simulink model "project_model_UPDATE"  (R2020a)
settings: Solver=FixedStepAuto  StartTime=0.0  StopTime=10.0  FixedStep=1e-3  RelTol=1e-3  EnableMultiTasking=on
undefined symbols (not defined in the file): D0, D1, D10, D11, D12, D13, D2, D3, D4, D5, D6, D7, D8, D9, PTA0, PTA1, PTA2, PTB23, PTB9, PTC16, PTC17, PTC2, PTC3, PTC4, PTD0, PTD1, PTD2, PTD3
libraries: frdmk64flib x15
settings Model: ExtModeTrigDuration=5  Creator=harry  LastModifiedBy=harry
settings OptimizationCC: EnhancedBackFolding=on  PassReuseOutputArgsAs=Individual arguments  ZeroExternalMemoryAtStartup=off  ZeroInternalMemoryAtStartup=off  MaxStackSize=64  OptimizeBlockOrder=speed  DifferentSizesBufferReuse=on  OptimizationCustomize=off  EfficientTunableParamExpr=on
settings DebuggingCC: ParameterTunabilityLossMsg=error  UnconnectedInputMsg=none  UnconnectedOutputMsg=none  UnconnectedLineMsg=none  SFMachineParentedDataDiag=error
settings HardwareCC: ProdBitPerPointer=32  ProdBitPerSizeT=32  ProdBitPerPtrDiffT=32  ProdLargestAtomicInteger=Long  ProdLargestAtomicFloat=Double  ProdWordSize=32  ProdHWDeviceType=ARM Compatible->ARM Cortex
settings SFSimCC: MATLABDynamicMemAlloc=off
settings RTWCC: SystemTargetFile=ert.tlc  HardwareBoard=NXP FRDM-K64F  TemplateMakefile=ert_default_tmf  Toolchain=GNU Tools for ARM Embedded Processors
settings CodeAppCC: ForceParamTrailComments=on  IgnoreCustomStorageClasses=off  OperatorAnnotations=on  SimulinkDataObjDesc=on  SFDataObjDesc=on  InsertBlockDesc=on
settings ERTTargetCC: ExtModeTransport=4  ExtModeMexFile=sendToCommService

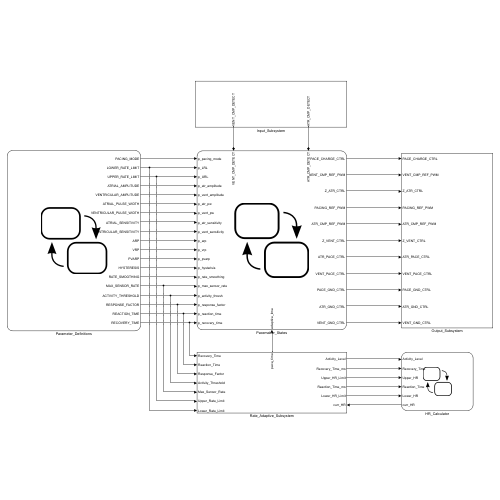
[thumbnail: Simulink's stored preview of the top-level diagram]
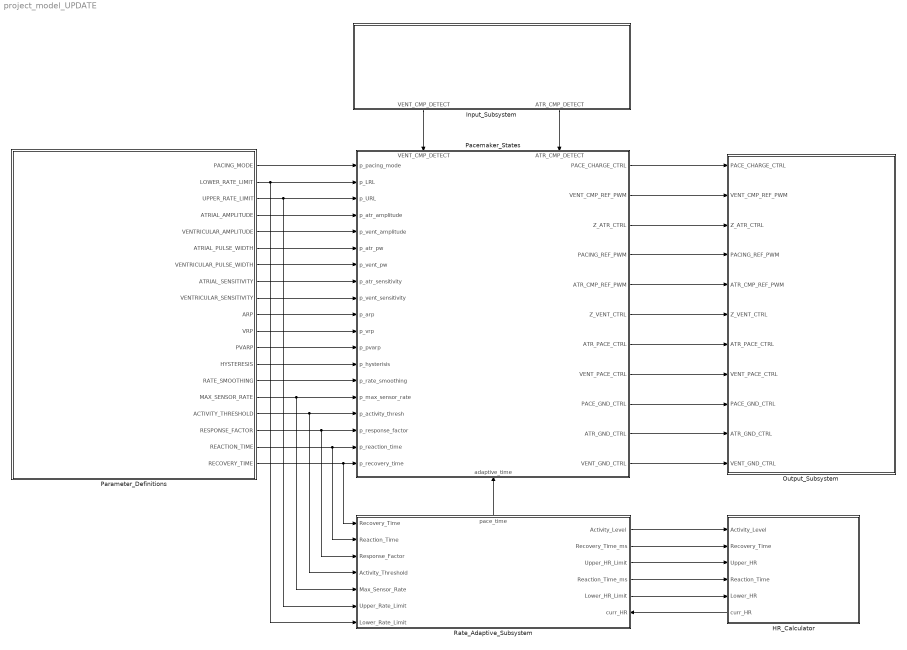
== system project_model_UPDATE ==
  HR_Calculator : Stateflow chart  TreatAsAtomicUnit=on
      settings: PortSchema="{\"entries\":[{\"content\":{\"sides\":[{\"content\":{\"connectorIds\":[\"In5\",\"In2\",\"In3\",\"In4\",\"In1\",\"Out1\"]},\"type\":\"ConnectorPlacement.EquallySpacedRectSide\",\"uuid\":\"4fd71a97-0d96-44cf-9a3b-b475d577ae04\"},{\"content\":{\"connectorIds\":[],\"side\":\"RIGHT\"},\"type\":\"ConnectorPlacement.EquallySpacedRectSide\",\"uuid\":\"faba256d-fac9-4ab5-bd75-12f2978d4ab7\"},{\"content\":{\"connectorIds\":[],\"side\":\"TOP\"},\"type\":\"ConnectorPlacement.EquallySpacedRectSide\",\"uuid\":\"a02d704a-be11-4cb0-b416-0f22440acd8a\"}]},\"type\":\"ConnectorPlacement.EquallySpacedConnector\",\"uuid\":\"fcc24184-24f4-4090-bbbe-791745e2298d\"}],\"packageUris\":[\"http://schema.mathworks.com/mf0/Connector/R2020b\"],\"version\":\"1.0\"}"
  Input_Subsystem : Subsystem
      settings: PortSchema="{\"entries\":[{\"content\":{\"sides\":[{\"content\":{\"connectorIds\":[]},\"type\":\"ConnectorPlacement.EquallySpacedRectSide\",\"uuid\":\"7aa35272-78af-4b86-b792-d4552822e5cd\"},{\"content\":{\"connectorIds\":[],\"side\":\"RIGHT\"},\"type\":\"ConnectorPlacement.EquallySpacedRectSide\",\"uuid\":\"1eeedbdd-e182-4d72-ab10-92c9b2e47973\"},{\"content\":{\"connectorIds\":[],\"side\":\"TOP\"},\"type\":\"ConnectorPlacement.EquallySpacedRectSide\",\"uuid\":\"983587ba-d25a-459a-9a3e-9f5267716506\"},{\"content\":{\"connectorIds\":[\"Out1\",\"Out2\"],\"side\":\"BOTTOM\"},\"type\":\"ConnectorPlacement.EquallySpacedRectSide\",\"uuid\":\"0cdd1530-a104-439a-8a9c-6ed3bc5e5b37\"}]},\"type\":\"ConnectorPlacement.EquallySpacedConnector\",\"uuid\":\"2c1020c0-9cac-4181-8f0f-8201f6fe3f1b\"}],\"packageUris\":[\"http://schema.mathworks.com/mf0/Connector/R2020b\"],\"version\":\"1.0\"}"
  Output_Subsystem : Subsystem
  Pacemaker_States : Stateflow chart  TreatAsAtomicUnit=on
      settings: PortSchema="{\"entries\":[{\"content\":{\"sides\":[{\"content\":{\"connectorIds\":[\"In9\",\"In5\",\"In15\",\"In7\",\"In4\",\"In8\",\"In6\",\"In13\",\"In14\",\"In11\",\"In12\",\"In17\",\"In10\",\"In16\",\"In18\",\"In19\",\"In20\",\"In22\",\"In21\"]},\"type\":\"ConnectorPlacement.EquallySpacedRectSide\",\"uuid\":\"f7c19d4e-8469-492c-a227-d3ddaf8b11c5\"},{\"content\":{\"connectorIds\":[\"Out8\",\"Out10\",\"Out1\",\"Out7\",\"Out11\",\"Out2\",\"Out3\",\"Out4\",\"Out9\",\"Out5\",\"Out6\"],\"side\":\"RIGHT\"},\"type\":\"ConnectorPlacement.EquallySpacedRectSide\",\"uuid\":\"dec5cef5-f41f-4673-aab9-f0ca8e60eeee\"},{\"content\":{\"connectorIds\":[\"In2\",\"In3\"],\"side\":\"TOP\"},\"type\":\"ConnectorPlacement.EquallySpacedRectSide\",\"uuid\":\"d69c500f-a27d-47d0-a981-29ab2c08cb35\"},{\"content\":{\"connectorIds\":[\"In1\"],\"side\":\"BOTTOM\"},\"type\":\"ConnectorPlacement.EquallySpacedRectSide\",\"uuid\":\"de5bd18b-94e5-479b-a57c-c3af68974efa\"}]},\"type\":\"ConnectorPlacement.EquallySpacedConnector\",\"uuid\":\"10b708de-b80e-4994-a949-6ddae67c2dfd\"}],\"packageUris\":[\"http://schema.mathworks.com/mf0/Connector/R2020b\"],\"version\":\"1.0\"}"
  Parameter_Definitions : Stateflow chart  TreatAsAtomicUnit=on
      settings: PortSchema="{\"entries\":[{\"content\":{\"sides\":[{\"content\":{\"connectorIds\":[]},\"type\":\"ConnectorPlacement.EquallySpacedRectSide\",\"uuid\":\"6604c324-2550-41c6-b2f2-71f3c706ced3\"},{\"content\":{\"connectorIds\":[\"Out1\",\"Out2\",\"Out3\",\"Out4\",\"Out7\",\"Out5\",\"Out9\",\"Out8\",\"Out6\",\"Out14\",\"Out13\",\"Out12\",\"Out11\",\"Out10\",\"Out16\",\"Out19\",\"Out15\",\"Out17\",\"Out18\"],\"side\":\"RIGHT\"},\"type\":\"ConnectorPlacement.EquallySpacedRectSide\",\"uuid\":\"7ef386a9-7013-4033-b302-df52cb7a11b5\"},{\"content\":{\"connectorIds\":[],\"side\":\"TOP\"},\"type\":\"ConnectorPlacement.EquallySpacedRectSide\",\"uuid\":\"6c75a8fc-d552-4f9b-9a9a-6aef7cb72f4d\"}]},\"type\":\"ConnectorPlacement.EquallySpacedConnector\",\"uuid\":\"c0dbf2bf-9097-47f1-93b4-de483c75bb4c\"}],\"packageUris\":[\"http://schema.mathworks.com/mf0/Connector/R2020b\"],\"version\":\"1.0\"}"
  Rate_Adaptive_Subsystem : Subsystem
      settings: PortSchema="{\"entries\":[{\"content\":{\"sides\":[{\"content\":{\"connectorIds\":[\"In1\",\"In2\",\"In3\",\"In4\",\"In5\",\"In6\",\"In7\"]},\"type\":\"ConnectorPlacement.EquallySpacedRectSide\",\"uuid\":\"0e73cd95-fd23-47fa-82ad-61e0ef758ad8\"},{\"content\":{\"connectorIds\":[\"Out1\",\"Out2\",\"Out3\",\"Out4\",\"Out5\",\"In8\"],\"side\":\"RIGHT\"},\"type\":\"ConnectorPlacement.EquallySpacedRectSide\",\"uuid\":\"257d0885-109f-47f8-9bd4-99d2095959ba\"},{\"content\":{\"connectorIds\":[\"Out6\"],\"side\":\"TOP\"},\"type\":\"ConnectorPlacement.EquallySpacedRectSide\",\"uuid\":\"5fbd8ae3-cd68-4bdc-a329-22cd7db730ea\"}]},\"type\":\"ConnectorPlacement.EquallySpacedConnector\",\"uuid\":\"229e8082-3f61-43cc-9449-39b4152275b7\"}],\"packageUris\":[\"http://schema.mathworks.com/mf0/Connector/R2020b\"],\"version\":\"1.0\"}"
  wires:
  Parameter_Definitions/10(RATE_SMOOTHING) -> Pacemaker_States/16(p_rate_smoothing)
  Parameter_Definitions/2(LOWER_RATE_LIMIT) -> Rate_Adaptive_Subsystem/7(Lower_Rate_Limit), Pacemaker_States/5(p_LRL)
  Rate_Adaptive_Subsystem/5(Lower_HR_Limit) -> HR_Calculator/1(Lower_HR)
  Parameter_Definitions/18(RECOVERY_TIME) -> Rate_Adaptive_Subsystem/1(Recovery_Time), Pacemaker_States/21(p_recovery_time)
  Pacemaker_States/9(PACE_GND_CTRL) -> Output_Subsystem/9(PACE_GND_CTRL)
  Parameter_Definitions/14(ARP) -> Pacemaker_States/11(p_arp)
  Pacemaker_States/5(ATR_GND_CTRL) -> Output_Subsystem/10(ATR_GND_CTRL)
  Pacemaker_States/10(VENT_CMP_REF_PWM) -> Output_Subsystem/2(VENT_CMP_REF_PWM)
  Pacemaker_States/6(VENT_GND_CTRL) -> Output_Subsystem/11(VENT_GND_CTRL)
  Parameter_Definitions/11(HYSTERESIS) -> Pacemaker_States/10(p_hysterisis)
  Rate_Adaptive_Subsystem/2(Recovery_Time_ms) -> HR_Calculator/2(Recovery_Time)
  Input_Subsystem/1(VENT_CMP_DETECT) -> Pacemaker_States/2(VENT_CMP_DETECT)
  Rate_Adaptive_Subsystem/6(pace_time) -> Pacemaker_States/1(adaptive_time)
  HR_Calculator/1(curr_HR) -> Rate_Adaptive_Subsystem/8(curr_HR)
  Input_Subsystem/2(ATR_CMP_DETECT) -> Pacemaker_States/3(ATR_CMP_DETECT)
  Pacemaker_States/8(PACE_CHARGE_CTRL) -> Output_Subsystem/1(PACE_CHARGE_CTRL)
  Rate_Adaptive_Subsystem/4(Reaction_Time_ms) -> HR_Calculator/4(Reaction_Time)
  Parameter_Definitions/5(ATRIAL_PULSE_WIDTH) -> Pacemaker_States/8(p_atr_pw)
  Parameter_Definitions/7(VENTRICULAR_AMPLITUDE) -> Pacemaker_States/4(p_vent_amplitude)
  Parameter_Definitions/4(ATRIAL_AMPLITUDE) -> Pacemaker_States/7(p_atr_amplitude)
  Pacemaker_States/11(ATR_CMP_REF_PWM) -> Output_Subsystem/5(ATR_CMP_REF_PWM)
  Parameter_Definitions/6(VENTRICULAR_SENSITIVITY) -> Pacemaker_States/14(p_vent_sensitivity)
  Parameter_Definitions/19(ACTIVITY_THRESHOLD) -> Rate_Adaptive_Subsystem/4(Activity_Threshold), Pacemaker_States/19(p_activity_thresh)
  Parameter_Definitions/17(REACTION_TIME) -> Rate_Adaptive_Subsystem/2(Reaction_Time), Pacemaker_States/22(p_reaction_time)
  Parameter_Definitions/13(VRP) -> Pacemaker_States/12(p_vrp)
  Rate_Adaptive_Subsystem/1(Activity_Level) -> HR_Calculator/5(Activity_Level)
  Parameter_Definitions/1(PACING_MODE) -> Pacemaker_States/9(p_pacing_mode)
  Rate_Adaptive_Subsystem/3(Upper_HR_Limit) -> HR_Calculator/3(Upper_HR)
  Parameter_Definitions/12(PVARP) -> Pacemaker_States/17(p_pvarp)
  Parameter_Definitions/16(MAX_SENSOR_RATE) -> Rate_Adaptive_Subsystem/5(Max_Sensor_Rate), Pacemaker_States/18(p_max_sensor_rate)
  Parameter_Definitions/9(VENTRICULAR_PULSE_WIDTH) -> Pacemaker_States/6(p_vent_pw)
  Pacemaker_States/3(ATR_PACE_CTRL) -> Output_Subsystem/7(ATR_PACE_CTRL)
  Pacemaker_States/7(PACING_REF_PWM) -> Output_Subsystem/4(PACING_REF_PWM)
  Pacemaker_States/4(VENT_PACE_CTRL) -> Output_Subsystem/8(VENT_PACE_CTRL)
  Parameter_Definitions/15(RESPONSE_FACTOR) -> Rate_Adaptive_Subsystem/3(Response_Factor), Pacemaker_States/20(p_response_factor)
  Parameter_Definitions/3(UPPER_RATE_LIMIT) -> Rate_Adaptive_Subsystem/6(Upper_Rate_Limit), Pacemaker_States/15(p_URL)
  Pacemaker_States/1(Z_ATR_CTRL) -> Output_Subsystem/3(Z_ATR_CTRL)
  Pacemaker_States/2(Z_VENT_CTRL) -> Output_Subsystem/6(Z_VENT_CTRL)
  Parameter_Definitions/8(ATRIAL_SENSITIVITY) -> Pacemaker_States/13(p_atr_sensitivity)

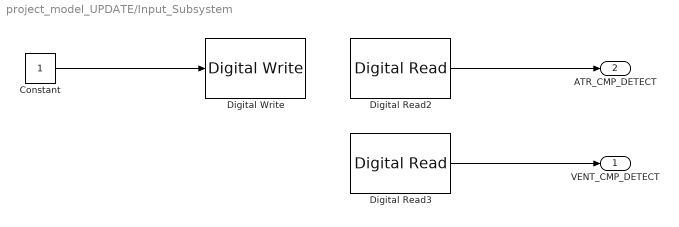
== system project_model_UPDATE/Input_Subsystem ==
  Constant : Constant
  Digital Read2 : frdmk64flib/Digital Read  Whichpin=PTC16 (D0)  SampleTime=-1
  Digital Read3 : frdmk64flib/Digital Read  Whichpin=PTC17 (D1)  SampleTime=-1
  Digital Write : frdmk64flib/Digital Write  Whichpin=PTD1 (D13)
  VENT_CMP_DETECT : Outport
  ATR_CMP_DETECT : Outport  Port=2
  wires:
  Constant/1 -> Digital Write/1
  Digital Read2/1 -> ATR_CMP_DETECT/1
  Digital Read3/1 -> VENT_CMP_DETECT/1

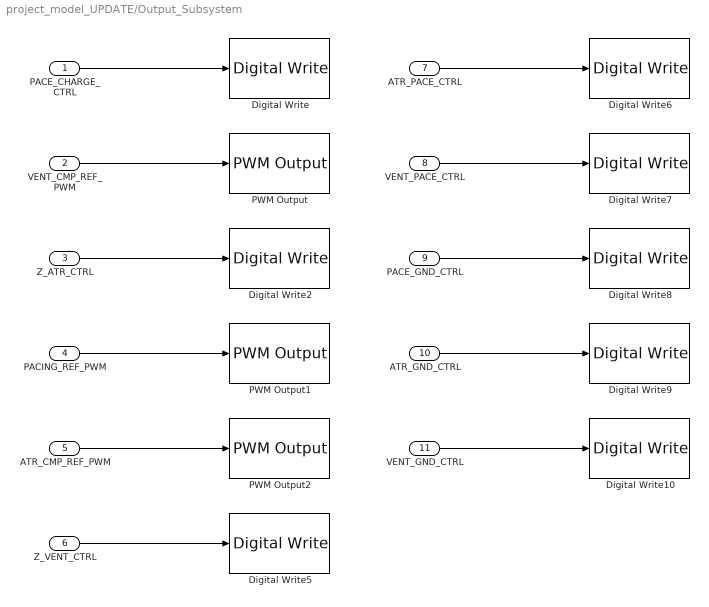
== system project_model_UPDATE/Output_Subsystem ==
  PACE_CHARGE_CTRL : Inport
  VENT_CMP_REF_PWM : Inport  Port=2
  Z_ATR_CTRL : Inport  Port=3
  PACING_REF_PWM : Inport  Port=4
  ATR_CMP_REF_PWM : Inport  Port=5
  Z_VENT_CTRL : Inport  Port=6
  ATR_PACE_CTRL : Inport  Port=7
  VENT_PACE_CTRL : Inport  Port=8
  PACE_GND_CTRL : Inport  Port=9
  ATR_GND_CTRL : Inport  Port=10
  VENT_GND_CTRL : Inport  Port=11
  Digital Write : frdmk64flib/Digital Write  Whichpin=PTB9 (D2)
  Digital Write10 : frdmk64flib/Digital Write  Whichpin=PTD3 (D12)
  Digital Write2 : frdmk64flib/Digital Write  Whichpin=PTB23 (D4)
  Digital Write5 : frdmk64flib/Digital Write  Whichpin=PTC3 (D7)
  Digital Write6 : frdmk64flib/Digital Write  Whichpin=PTA0 (D8)
  Digital Write7 : frdmk64flib/Digital Write  Whichpin=PTC4 (D9)
  Digital Write8 : frdmk64flib/Digital Write  Whichpin=PTD0 (D10)
  Digital Write9 : frdmk64flib/Digital Write  Whichpin=PTD2 (D11)
  PWM Output : frdmk64flib/PWM Output  Whichpin=PTA1 (D3)  InitialFrequency=2000  InitialDutyCycle=0
  PWM Output1 : frdmk64flib/PWM Output  Whichpin=PTA2 (D5)  InitialFrequency=2000  InitialDutyCycle=0
  PWM Output2 : frdmk64flib/PWM Output  Whichpin=PTC2 (D6)  InitialFrequency=2000  InitialDutyCycle=0
  wires:
  PACE_CHARGE_CTRL/1 -> Digital Write/1
  VENT_CMP_REF_PWM/1 -> PWM Output/1
  Z_ATR_CTRL/1 -> Digital Write2/1
  ATR_CMP_REF_PWM/1 -> PWM Output2/1
  Z_VENT_CTRL/1 -> Digital Write5/1
  PACING_REF_PWM/1 -> PWM Output1/1
  VENT_PACE_CTRL/1 -> Digital Write7/1
  ATR_GND_CTRL/1 -> Digital Write9/1
  PACE_GND_CTRL/1 -> Digital Write8/1
  ATR_PACE_CTRL/1 -> Digital Write6/1
  VENT_GND_CTRL/1 -> Digital Write10/1

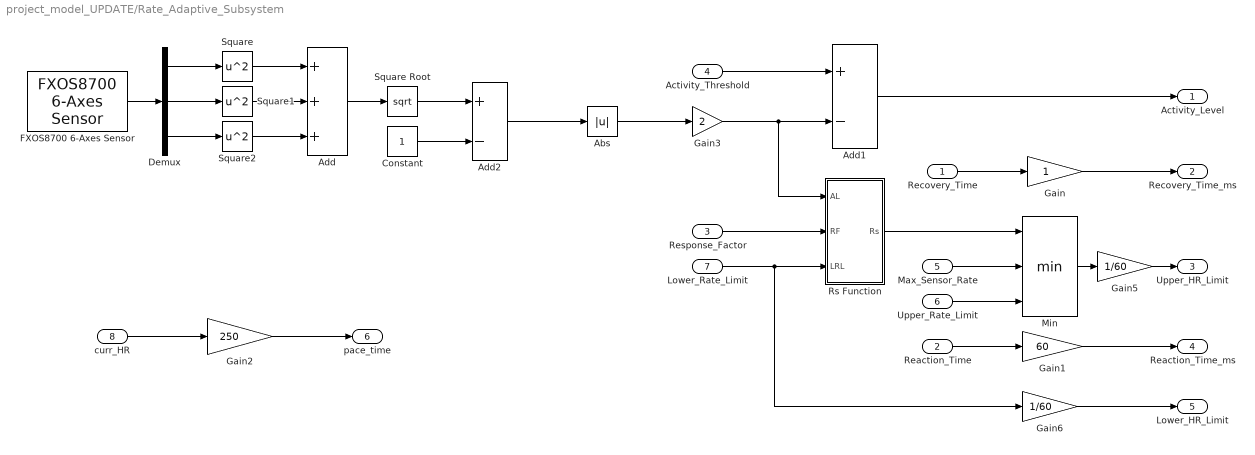
== system project_model_UPDATE/Rate_Adaptive_Subsystem ==
  Recovery_Time : Inport
  Reaction_Time : Inport  Port=2
  Response_Factor : Inport  Port=3
  Activity_Threshold : Inport  Port=4
  Max_Sensor_Rate : Inport  Port=5
  Upper_Rate_Limit : Inport  Port=6
  Lower_Rate_Limit : Inport  Port=7
  curr_HR : Inport  Port=8
  Abs : Abs
  Add : Sum  Inputs=+++
  Add1 : Sum  Inputs=+-
  Add2 : Sum  Inputs=+-
  Constant : Constant
  Demux : Demux  Outputs=3
  FXOS8700 6-Axes Sensor : frdmk64flib/FXOS8700 6-Axes Sensor  Activesensor=Accelerometer only  ODR=800Hz  HybridODR=400Hz  Accelfullrange=-4g to +4g  SampleTime=-1
  Gain : Gain
  Gain1 : Gain  Gain=60
  Gain2 : Gain  Gain=250
  Gain3 : Gain  Gain=2
  Gain5 : Gain  Gain=1/60
  Gain6 : Gain  Gain=1/60
  Min : MinMax  Inputs=3
  Rs Function : MATLAB Function  TreatAsAtomicUnit=on
  Square : Math  Operator=square  SaturateOnIntegerOverflow=on
  Square Root : Sqrt  SaturateOnIntegerOverflow=on
  Square1 : Math  Operator=square  SaturateOnIntegerOverflow=on
  Square2 : Math  Operator=square  SaturateOnIntegerOverflow=on
  Activity_Level : Outport
  Recovery_Time_ms : Outport  Port=2
  Upper_HR_Limit : Outport  Port=3
  Reaction_Time_ms : Outport  Port=4
  Lower_HR_Limit : Outport  Port=5
  pace_time : Outport  Port=6
  wires:
  FXOS8700 6-Axes Sensor/1 -> Demux/1
  Demux/1 -> Square/1
  Demux/2 -> Square1/1
  Demux/3 -> Square2/1
  Square1/1 -> Add/2
  Square/1 -> Add/1
  Square2/1 -> Add/3
  Add/1 -> Square Root/1
  Lower_Rate_Limit/1 -> Gain6/1, Rs Function/3(LRL)
  Response_Factor/1 -> Rs Function/2(RF)
  Max_Sensor_Rate/1 -> Min/2
  Rs Function/1(Rs) -> Min/1
  Activity_Threshold/1 -> Add1/1
  Add1/1 -> Activity_Level/1
  Recovery_Time/1 -> Gain/1
  Reaction_Time/1 -> Gain1/1
  Gain/1 -> Recovery_Time_ms/1
  Gain1/1 -> Reaction_Time_ms/1
  Gain2/1 -> pace_time/1
  Gain3/1 -> Rs Function/1(AL), Add1/2
  Square Root/1 -> Add2/1
  Constant/1 -> Add2/2
  Add2/1 -> Abs/1
  Abs/1 -> Gain3/1
  Upper_Rate_Limit/1 -> Min/3
  curr_HR/1 -> Gain2/1
  Gain6/1 -> Lower_HR_Limit/1
  Gain5/1 -> Upper_HR_Limit/1
  Min/1 -> Gain5/1

== stateflow chart project_model_UPDATE/Parameter_Definitions ==
  state Parameter_Definitions
    entry:
    %Defining the initial paramater values
    PACING_MODE = 7;
    LOWER_RATE_LIMIT = 60;
    UPPER_RATE_LIMIT = 120;
    ATRIAL_AMPLITUDE = 3500;
    VENTRICULAR_AMPLITUDE = 5000;
    ATRIAL_PULSE_WIDTH = 0.4;
    VENTRICULAR_PULSE_WIDTH = 0.4;
    ATRIAL_SENSITIVITY = 2.75;
    VENTRICULAR_SENSITIVITY = 2.5;
    ARP = 500;
    VRP = 320;
    PVARP = 250;
    HYSTERESIS = false;
    RATE_SMOOTHING = false;
    MAX_SENSOR_RATE = 120;
    ACTIVITY_THRESHOLD = 5;
    RESPONSE_FACTOR = 8;
    REACTION_TIME = 10;
    RECOVERY_TIME = 8;
  (default) -> Parameter_Definitions
  data: PACING_MODE output; LOWER_RATE_LIMIT output; UPPER_RATE_LIMIT output; ATRIAL_AMPLITUDE output; ATRIAL_PULSE_WIDTH output; VENTRICULAR_SENSITIVITY output; VENTRICULAR_AMPLITUDE output; ATRIAL_SENSITIVITY output; VENTRICULAR_PULSE_WIDTH output; RATE_SMOOTHING output; HYSTERESIS output; PVARP output; VRP output; ARP output; RESPONSE_FACTOR output; MAX_SENSOR_RATE output; REACTION_TIME output; RECOVERY_TIME output; ACTIVITY_THRESHOLD output

== matlab function project_model_UPDATE/Rate_Adaptive_Subsystem/Rs Function ==
  data: AL input; RF input; Rs output; LRL input
function Rs = fcn(AL, RF , LRL)

Rs = LRL + 4*RF*exp(AL+1);

== stateflow chart project_model_UPDATE/Pacemaker_States ==
  state VOOR
    entry:
    state Initial_VOOR
      entry:
      %This is the initial state to define
      %varriables that wont change
      VOOR_amp = (p_vent_amplitude/5000)*100;
      ATR_PACE_CTRL=0;
      ATR_GND_CTRL= 0;
      Z_ATR_CTRL=0;
      Z_VENT_CTRL=0;
    state Discharge_VOOR
      entry:
      %pacing state 3
      PACE_GND_CTRL=1;
      VENT_PACE_CTRL=0;
      VENT_GND_CTRL=1;
      %pacing state 1
      PACING_REF_PWM= VOOR_amp;
      PACE_CHARGE_CTRL=1;
    state Charge_VOOR
      entry:
      %pacing state 2
      PACE_CHARGE_CTRL=0;
      PACE_GND_CTRL=1;
      VENT_GND_CTRL=0;
      VENT_PACE_CTRL=1;
    (default) -> Initial_VOOR
    Initial_VOOR -> Discharge_VOOR
    Discharge_VOOR -> Charge_VOOR : [after(adaptive_time - p_vent_pw, msec)]
    Charge_VOOR -> Discharge_VOOR : [after(p_vent_pw, msec)]
  state VOO
    entry:
    state Discharge_VOO
      entry:
      %pacing state 3
      PACE_GND_CTRL=1;
      VENT_PACE_CTRL=0;
      VENT_GND_CTRL=1;
      %pacing state 1
      PACING_REF_PWM= VOO_amp;
      PACE_CHARGE_CTRL=1;
    state Initial_VOO
      entry:
      %This is the initial state to define
      %varriables that wont change
      discharge_time = ((p_LRL/60)*1000)-p_vent_pw;
      VOO_amp = (p_vent_amplitude/5000)*100;
      ATR_PACE_CTRL=0;
      ATR_GND_CTRL= 0;
      Z_ATR_CTRL=0;
      Z_VENT_CTRL=0;
    state Charge_VOO
      entry:
      %pacing state 2
      PACE_CHARGE_CTRL=0;
      PACE_GND_CTRL=1;
      VENT_GND_CTRL=0;
      VENT_PACE_CTRL=1;
    (default) -> Initial_VOO
    Initial_VOO -> Discharge_VOO
    Discharge_VOO -> Charge_VOO : [after(discharge_time, msec)]
    Charge_VOO -> Discharge_VOO : [after(p_vent_pw, msec)]
  state AOO
    entry:
    state Discharge_AOO
      entry:
      %pacing state 3
      PACE_GND_CTRL=1;
      ATR_PACE_CTRL=0;
      ATR_GND_CTRL=1;
      %pacing state 1
      PACING_REF_PWM= AOO_amp;
      PACE_CHARGE_CTRL=1;
    state Initial_AOO
      entry:
      %Defining variables
      discharge_time = ((60/p_LRL)*1000)-p_atr_pw;
      AOO_amp = (p_atr_amplitude/5000)*100;
      Z_VENT_CTRL=0;
      VENT_GND_CTRL=0;
      VENT_PACE_CTRL=0;
      Z_ATR_CTRL=0;
    state Charge_AOO
      entry:
      %pacing state 2
      PACE_CHARGE_CTRL=0;
      PACE_GND_CTRL=1;
      ATR_GND_CTRL= 0;
      ATR_PACE_CTRL=1;
    (default) -> Initial_AOO
    Initial_AOO -> Discharge_AOO
    Discharge_AOO -> Charge_AOO : [after(discharge_time, msec)]
    Charge_AOO -> Discharge_AOO : [after(p_atr_pw, msec)]
  state Initial_State
    entry:
    VENT_CMP_REF_PWM = 52;
    ATR_CMP_REF_PWM = 51;
  state VVIR
    entry:
    state Discharge_VVI
      entry:
      %pacing state 3
      PACE_GND_CTRL=1;
      VENT_PACE_CTRL=0;
      VENT_GND_CTRL=1;
      % pacing state 1
      PACING_REF_PWM= VVIR_amp;
      PACE_CHARGE_CTRL=1;
    state Initial_VVIR
      entry:
      %Initial state defining variables
      VVIR_amp = (p_vent_amplitude/5000)*100;
      ATR_PACE_CTRL=0;
      ATR_GND_CTRL= 0;
      Z_ATR_CTRL=0;
      Z_VENT_CTRL=0;
    state Charge_VVIR
      entry:
      %pacing state 2
      PACE_CHARGE_CTRL=0;
      PACE_GND_CTRL=1;
      VENT_GND_CTRL=0;
      VENT_PACE_CTRL=1;
    (default) -> Initial_VVIR
    Initial_VVIR -> VVIR.Discharge_VVI
    VVIR.Discharge_VVI -> (junction 132)
    (junction 132) -> VVIR.Discharge_VVI [order 2] : [VENT_CMP_DETECT == true]
    Charge_VVIR -> VVIR.Discharge_VVI : [after(p_vent_pw, msec)]
    (junction 132) -> Charge_VVIR [order 1] : [after(adaptive_time - p_vent_pw, msec) && VENT_CMP_DETECT == false]
  state AOOR
    entry:
    state Discharge_AOOR
      entry:
      %pacing state 3
      PACE_GND_CTRL=1;
      ATR_PACE_CTRL=0;
      ATR_GND_CTRL=1;
      %pacing state 1
      PACING_REF_PWM= AOOR_amp;
      PACE_CHARGE_CTRL=1;
    state Initial_AOOR
      entry:
      %Defining variables
      AOOR_amp = (p_atr_amplitude/5000)*100;
      Z_VENT_CTRL=0;
      VENT_GND_CTRL=0;
      VENT_PACE_CTRL=0;
      Z_ATR_CTRL=0;
    state Charge_AOOR
      entry:
      %pacing state 2
      PACE_CHARGE_CTRL=0;
      PACE_GND_CTRL=1;
      ATR_GND_CTRL= 0;
      ATR_PACE_CTRL=1;
    (default) -> Initial_AOOR
    Initial_AOOR -> Discharge_AOOR
    Charge_AOOR -> Discharge_AOOR : [after(p_atr_pw, msec)]
    Discharge_AOOR -> Charge_AOOR : [after(adaptive_time - p_atr_pw, msec)]
  state VVI
    entry:
    state Discharge_VVI
      entry:
      %pacing state 3
      PACE_GND_CTRL=1;
      VENT_PACE_CTRL=0;
      VENT_GND_CTRL=1;
      % pacing state 1
      PACING_REF_PWM= VVI_amp;
      PACE_CHARGE_CTRL=1;
    state Initial_VVI
      entry:
      %Initial state defining variables
      discharge_time = ((60/p_LRL)*1000)-p_vent_pw;
      VVI_amp = (p_vent_amplitude/5000)*100;
      ATR_PACE_CTRL=0;
      ATR_GND_CTRL= 0;
      Z_ATR_CTRL=0;
      Z_VENT_CTRL=0;
    state Charge_VVI
      entry:
      %pacing state 2
      PACE_CHARGE_CTRL=0;
      PACE_GND_CTRL=1;
      VENT_GND_CTRL=0;
      VENT_PACE_CTRL=1;
    (default) -> Initial_VVI
    Initial_VVI -> VVI.Discharge_VVI
    VVI.Discharge_VVI -> (junction 38)
    Charge_VVI -> VVI.Discharge_VVI : [after(p_vent_pw, msec)]
    (junction 38) -> VVI.Discharge_VVI [order 2] : [VENT_CMP_DETECT == true]
    (junction 38) -> Charge_VVI [order 1] : [after(discharge_time, msec) && VENT_CMP_DETECT == false]
  state AAI
    entry:
    state Discharge_AAI
      entry:
      %pacing state 3
      PACE_GND_CTRL=1;
      ATR_PACE_CTRL=0;
      ATR_GND_CTRL=1;
      %pacing state 1
      PACING_REF_PWM= AAI_amp;
      PACE_CHARGE_CTRL=1;
    state Initial_AAI
      entry:
      %initial state defining variables
      discharge_time = ((60/p_LRL)*1000)-p_atr_pw;
      AAI_amp = (p_atr_amplitude/5000)*100;
      Z_VENT_CTRL=0;
      VENT_GND_CTRL=0;
      VENT_PACE_CTRL=0;
      Z_ATR_CTRL=0;
    state Charge_AAI
      entry:
      %pacing state 2
      PACE_CHARGE_CTRL=0;
      PACE_GND_CTRL=1;
      ATR_GND_CTRL= 0;
      ATR_PACE_CTRL=1;
    (default) -> Initial_AAI
    Initial_AAI -> Discharge_AAI
    Discharge_AAI -> (junction 45)
    (junction 45) -> Discharge_AAI [order 2] : [ATR_CMP_DETECT == true]
    Charge_AAI -> Discharge_AAI : [after(p_atr_pw, msec)]
    (junction 45) -> Charge_AAI [order 1] : [after(discharge_time , msec) && ATR_CMP_DETECT == false]
  state AAIR
    entry:
    state Discharge_AAIR
      entry:
      %pacing state 3
      PACE_GND_CTRL=1;
      ATR_PACE_CTRL=0;
      ATR_GND_CTRL=1;
      %pacing state 1
      PACING_REF_PWM= AAIR_amp;
      PACE_CHARGE_CTRL=1;
    state Initial_AAIR
      entry:
      %initial state defining variables
      AAIR_amp = (p_atr_amplitude/5000)*100;
      Z_VENT_CTRL=0;
      VENT_GND_CTRL=0;
      VENT_PACE_CTRL=0;
      Z_ATR_CTRL=0;
    state Charge_AAIR
      entry:
      %pacing state 2
      PACE_CHARGE_CTRL=0;
      PACE_GND_CTRL=1;
      ATR_GND_CTRL= 0;
      ATR_PACE_CTRL=1;
    (default) -> Initial_AAIR
    Initial_AAIR -> Discharge_AAIR
    Discharge_AAIR -> (junction 117)
    (junction 117) -> Discharge_AAIR [order 2] : [ATR_CMP_DETECT == true]
    Charge_AAIR -> Discharge_AAIR : [after(p_atr_pw, msec)]
    (junction 117) -> Charge_AAIR [order 1] : [after(adaptive_time -p_atr_pw , msec) && ATR_CMP_DETECT == false]
  Initial_State -> VOOR [order 2] : [p_pacing_mode == 5]
  VOOR -> Initial_State : [p_pacing_mode ~= 5]
  VOO -> Initial_State : [p_pacing_mode ~= 1]
  AOO -> Initial_State : [p_pacing_mode ~= 2]
  Initial_State -> VOO [order 1] : [p_pacing_mode == 1]
  Initial_State -> AOO [order 6] : [p_pacing_mode == 2]
  (default) -> Initial_State
  AOOR -> Initial_State : [p_pacing_mode ~= 6]
  Initial_State -> VVIR [order 3] : [p_pacing_mode == 8]
  VVIR -> Initial_State : [p_pacing_mode ~=  8]
  Initial_State -> AOOR [order 5] : [p_pacing_mode == 6]
  Initial_State -> AAI [order 7] : [p_pacing_mode == 3]
  Initial_State -> VVI [order 8] : [p_pacing_mode == 4]
  VVI -> Initial_State : [p_pacing_mode ~=  4]
  AAIR -> Initial_State : [p_pacing_mode ~= 7]
  Initial_State -> AAIR [order 4] : [p_pacing_mode == 7]
  AAI -> Initial_State : [p_pacing_mode ~= 3]
  data: adaptive_time input; Z_ATR_CTRL output; Z_VENT_CTRL output; ATR_PACE_CTRL output; VENT_PACE_CTRL output; ATR_GND_CTRL output; VENT_GND_CTRL output; PACING_REF_PWM output; PACE_CHARGE_CTRL output; PACE_GND_CTRL output; VENT_CMP_REF_PWM output; ATR_CMP_REF_PWM output; VENT_CMP_DETECT input; ATR_CMP_DETECT input; p_vent_amplitude input; p_LRL input; p_vent_pw input; p_atr_amplitude input; p_atr_pw input; p_pacing_mode input; p_hysterisis input; p_arp input; p_vrp input; p_atr_sensitivity input; p_vent_sensitivity input; p_URL input; p_rate_smoothing input; p_pvarp input; discharge_time local; VOO_amp local; AOO_amp local; VVI_amp local; AAI_amp local; AOOR_amp local; AAIR_amp local; VVIR_amp local; p_max_sensor_rate input; p_activity_thresh input; p_response_factor input; p_recovery_time input; p_rp local; p_reaction_time input; curr_HR local; rate_slope local; p_curr_HR local; p_rs local; VOOR_amp local

== stateflow chart project_model_UPDATE/HR_Calculator ==
  state Maintain_Upper_Rate
    entry:
    curr_HR = Upper_HR;
  state Reaction_Rate_Definition
    entry:
    reaction_Rate = (Upper_HR - curr_HR)/Reaction_Time;
    curr_Level = Activity_Level;
  state Increase_HR
    entry:
    curr_HR = curr_HR + reaction_Rate *d_time
  state Entry_State
    entry:
    curr_HR = Lower_HR;
    reaction_Rate = (Upper_HR - Lower_HR)/Reaction_Time;
    recovery_Rate = (Lower_HR - Upper_HR)/Recovery_Time;
    curr_Level = Activity_Level;
    d_time = 0.1;
  state Decrease_HR
    entry:
    curr_HR = curr_HR + recovery_Rate *d_time
  state Define_Recovery_Rate
    entry:
    curr_Level = Activity_Level;
    recovery_Rate = (Lower_HR - curr_HR)/Recovery_Time;
  state Maintain_Lower_Rate
    entry:
    curr_HR = Lower_HR;
  Maintain_Upper_Rate -> (junction 25)
  (junction 19) -> Maintain_Upper_Rate [order 1] : [curr_HR >= Upper_HR]
  Reaction_Rate_Definition -> (junction 19)
  (junction 25) -> (junction 19) [order 2] : [Activity_Level == curr_Level ]{after(d_time, sec)}
  (junction 25) -> (junction 48) [order 1] : [Activity_Level ~= curr_Level ]
  Increase_HR -> (junction 25)
  (junction 19) -> Increase_HR [order 2]
  (junction 48) -> Reaction_Rate_Definition [order 2] : [Activity_Level > 0 ]{after(d_time,sec)}
  (default) -> Entry_State
  Entry_State -> (junction 48)
  (junction 32) -> (junction 48) [order 1] : [Activity_Level ~= curr_Level]
  (junction 48) -> Define_Recovery_Rate [order 1] : [Activity_Level <= 0]{after(d_time, sec)}
  (junction 35) -> Decrease_HR [order 2]
  Decrease_HR -> (junction 32)
  Define_Recovery_Rate -> (junction 35)
  (junction 32) -> (junction 35) [order 2] : [Activity_Level == curr_Level ]{after(d_time, sec)}
  Maintain_Lower_Rate -> (junction 32)
  (junction 35) -> Maintain_Lower_Rate [order 1] : [curr_HR <= Lower_HR]
  data: Lower_HR input; Recovery_Time input; Upper_HR input; Reaction_Time input; Activity_Level input; curr_HR output; recovery_Rate local; reaction_Rate local; curr_Level local; d_time local
